simulink model "PI_controller"  (R2013b)
settings: Solver=ode45  StartTime=0.0  StopTime=10.0  RelTol=1e-3
settings Model: Creator=training-it  LastModifiedBy=training-it

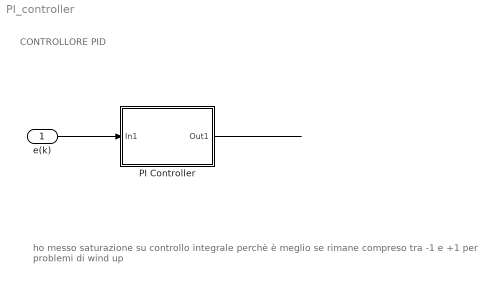
== system PI_controller ==
  note: ho messo saturazione su controllo integrale perchè è meglio se rimane compreso tra -1 e +1 per problemi di wind up
  note: CONTROLLORE PID
  e(k) : Inport
  PI Controller : Subsystem  mask{Ts=0.01, kp=0.3, ki=2}
      mask prompts: Ts "Sample Time"; kp "Guadagno Proporzionale"; ki "Guadagno Integrativo"
      mask init:
      | s1=['kp= ',num2str(kp)];
      | s2=['ki= ',num2str(ki)];
      | s=strvcat(s1,s2);  %sto concatenando verticalmente
      mask Display: disp(s)
  wires:
  e(k)/1 -> PI Controller/1(In1)
  PI Controller/1(Out1) -> ?

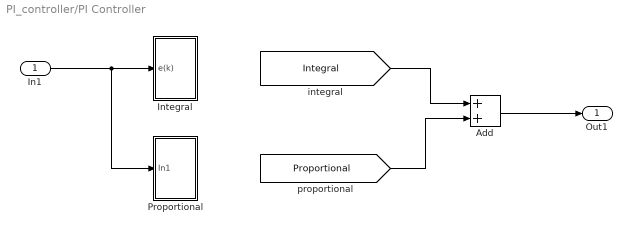
== system PI_controller/PI Controller ==
  In1 : Inport
  Add : Sum
  Integral : Subsystem
  Proportional : Subsystem
  Out1 : Outport
  wires:
  [Integral] -> Add/1
  Add/1 -> Out1/1
  In1/1 -> Proportional/1(In1), Integral/1(e(k))
  [Proportional] -> Add/2

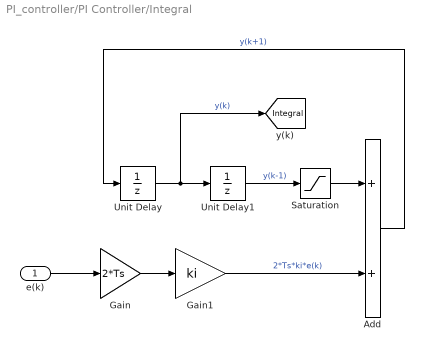
== system PI_controller/PI Controller/Integral ==
  e(k) : Inport
  Add : Sum
  Gain : Gain  Gain=2*Ts
  Gain1 : Gain  Gain=ki
  Saturation : Saturate  UpperLimit=1  LowerLimit=-1
      settings: AttributesFormatString=|
      | %<LowerLimit>
      | %<UpperLimit>
  Unit Delay : UnitDelay  SampleTime=Ts
  Unit Delay1 : UnitDelay  SampleTime=Ts
  tag scope: Integral=global
  wires:
  Gain1/1 -> Add/2  "2*Ts*ki*e(k)"
  Unit Delay/1 -> [Integral], Unit Delay1/1  "y(k)"
  Gain/1 -> Gain1/1
  Saturation/1 -> Add/1
  Unit Delay1/1 -> Saturation/1  "y(k-1)"
  e(k)/1 -> Gain/1
  Add/1 -> Unit Delay/1  "y(k+1)"

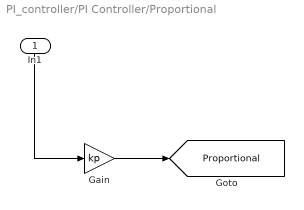
== system PI_controller/PI Controller/Proportional ==
  In1 : Inport
  Gain : Gain  Gain=kp
  tag scope: Proportional=global
  wires:
  Gain/1 -> [Proportional]
  In1/1 -> Gain/1
